simulink model "Sysmodel"  (R2020a)
settings: Solver=VariableStepAuto  StartTime=0.0  StopTime=1  RelTol=1e-3
values from neighbouring files (symbols this model uses):
  K_d = 2*z*wn/P_ball    [Ballplate.m]
  K_p = wn^2/P_ball    [Ballplate.m]
settings Model: Creator=surpe  LastModifiedBy=surpe

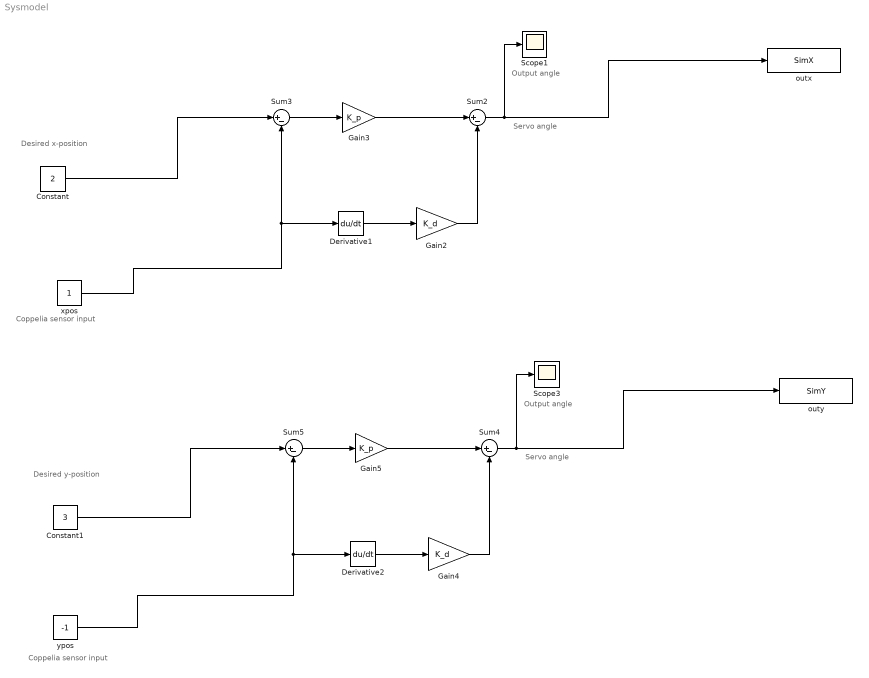
== system Sysmodel ==
  note: Output angle
  note: Desired x-position
  note: Coppelia sensor input
  note: Coppelia sensor input
  note: Output angle
  note: Servo angle
  note: Servo angle
  note: Desired y-position
  Constant : Constant  Value=2
  Constant1 : Constant  Value=3
  Derivative1 : Derivative
  Derivative2 : Derivative
  Gain2 : Gain  Gain=K_d
  Gain3 : Gain  Gain=K_p
  Gain4 : Gain  Gain=K_d
  Gain5 : Gain  Gain=K_p
  Scope1 : Scope
  Scope3 : Scope
  Sum{2..5} (4 alike) : Sum  Inputs=|+-
  outx : ToWorkspace  VariableName=SimX  SaveFormat=Timeseries  SampleTime=-1
  outy : ToWorkspace  VariableName=SimY  SaveFormat=Timeseries  SampleTime=-1
  xpos : Constant
  ypos : Constant  Value=-1
  wires:
  xpos/1 -> Sum3/2, Derivative1/1
  Gain5/1 -> Sum4/1
  Gain2/1 -> Sum2/2
  Sum3/1 -> Gain3/1
  Sum5/1 -> Gain5/1
  Constant1/1 -> Sum5/1
  ypos/1 -> Derivative2/1, Sum5/2
  Gain3/1 -> Sum2/1
  Derivative2/1 -> Gain4/1
  Constant/1 -> Sum3/1
  Gain4/1 -> Sum4/2
  Sum4/1 -> outy/1, Scope3/1
  Derivative1/1 -> Gain2/1
  Sum2/1 -> outx/1, Scope1/1
